simulink model "PulseGenerator_sim_2020"  (R2020b)
settings: Solver=ode4  StartTime=0.0  StopTime=2  FixedStep=0.05  RelTol=1e-3
settings Model: Creator=005274  LastModifiedBy=005274

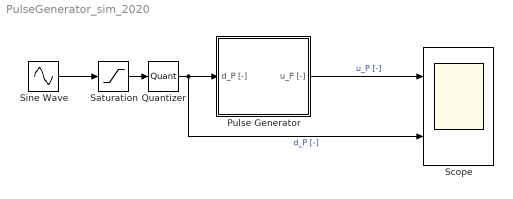
== system PulseGenerator_sim_2020 ==
  Pulse Generator : Subsystem  mask{n=1}
      mask prompts: n "bit"
  Quantizer : Quantizer  QuantizationInterval=1
  Saturation : Saturate  UpperLimit=255  LowerLimit=0
  Scope : Scope  NumInputPorts=2
  Sine Wave : Sin  Amplitude=255  Frequency=2*pi  SampleTime=0
  wires:
  Pulse Generator/1(u_P [-]) -> Scope/1  "u_P [-]"
  Quantizer/1 -> Scope/2, Pulse Generator/1(d_P [-])  "d_P [-]"
  Saturation/1 -> Quantizer/1
  Sine Wave/1 -> Saturation/1

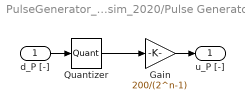
== system PulseGenerator_sim_2020/Pulse Generator ==
  d_P [-] : Inport
  Gain : Gain  Gain=200/(2^n-1)
  Quantizer : Quantizer  QuantizationInterval=1
  u_P [-] : Outport
  wires:
  Quantizer/1 -> Gain/1
  Gain/1 -> u_P [-]/1
  d_P [-]/1 -> Quantizer/1
